simulink model "parameter_estimation"  (R2021a)
settings: Solver=VariableStepAuto  StartTime=0.0  StopTime=time_est  RelTol=1e-3
values from neighbouring files (symbols this model uses):
  Delta = 0.04    [basic_imp_valid.m]    (also in battery_ekf.m = block.DialogPrm(1).Data; init_script.m = cur_est.Time(2)-cur_est.Time(1))
settings Model: Creator=saleh  LastModifiedBy=saleh

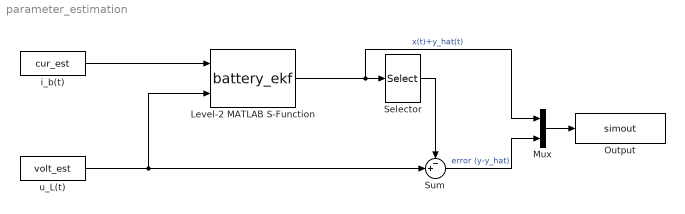
== system parameter_estimation ==
  Level-2 MATLAB S-Function : M-S-Function  FunctionName=battery_ekf  Parameters=Delta, x0, P0, a, Z_k, W_k, Qe
  Mux : Mux  Inputs=2
  Output : ToWorkspace  VariableName=simout  SampleTime=-1
  Selector : Selector  InputPortWidth=6  IndexOptions=Index vector (dialog)  Indices=[6]  OutputSizes=1
  Sum : Sum  Inputs=-+|
  i_b(t) : FromWorkspace  VariableName=cur_est  SampleTime=Delta
  u_L(t) : FromWorkspace  VariableName=volt_est  SampleTime=Delta
  wires:
  i_b(t)/1 -> Level-2 MATLAB S-Function/1
  u_L(t)/1 -> Sum/2, Level-2 MATLAB S-Function/2
  Level-2 MATLAB S-Function/1 -> Mux/1, Selector/1  "x(t)+y_hat(t)"
  Selector/1 -> Sum/1
  Sum/1 -> Mux/2  "error (y-y_hat)"
  Mux/1 -> Output/1
